simulink model "LQG_test"  (R2015a)
settings: Solver=ode5  StartTime=0.0  StopTime=14  FixedStep=1e-4  RelTol=1e-3
values from neighbouring files (symbols this model uses):
  Ak = [-64 -2560.5889522 8 186.2855092 1 -591.3291744 0 -1454.0827616 8 -3098.4577974 -142 -18500.7928836 ... (16 elements, 4x4)]    [controller.mat]    (also in main_matlab_step1.m = A-B*K-L*C)
  Ap = A(1:nn,1:nn)    [main_matlab_step1.m]    (also in plant.mat = [0 -330.46 0 -812.61 1 -12.15 0 -29.87 0 -2.44 0 -30.1 ... ()
  Bk = [64  -8; 2054  -280; -8  142; -1432  10169]    [controller.mat]    (also in main_matlab_step1.m = L)
  Bp = B    [main_matlab_step1.m]    (also in plant.mat = [0 2.71762 0 6.68268])
  Ck = [-64.81 -213.12 -1242.27 -85.82]    [controller.mat]    (also in main_matlab_step1.m = -K)
  Cp = C    [main_matlab_step1.m]    (also in plant.mat = [1  0  0  0; 0  0  1  0])
  Dk = [0 0]    [controller.mat]    (also in main_matlab_step1.m = zeros(1,2))
  Hp = H    [main_matlab_step1.m]    (also in plant.mat = [0 0 0 15.61])
libraries: simulink x1
settings Model: Creator=p4wp4w  LastModifiedBy=p4wp4w

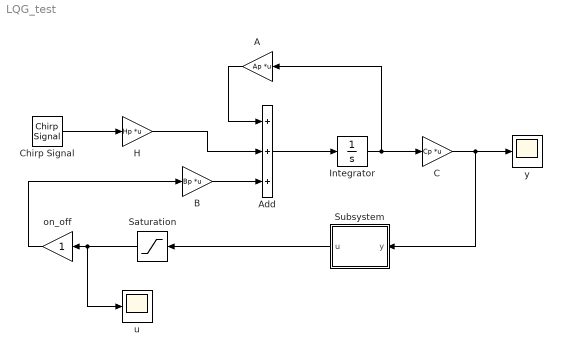
== system LQG_test ==
  A : Gain  Gain=Ap  Multiplication=Matrix(K*u)
  Add : Sum  Inputs=+++
  B : Gain  Gain=Bp  Multiplication=Matrix(K*u)
  C : Gain  Gain=Cp  Multiplication=Matrix(K*u)
  Chirp Signal : simulink/Sources/Chirp Signal  f1=0.1  T=14  f2=140
  H : Gain  Gain=Hp  Multiplication=Matrix(K*u)
  Integrator : Integrator
  Saturation : Saturate  UpperLimit=1.5  LowerLimit=-1.5
  Subsystem : Subsystem
  on_off : Gain
  u : Scope
      settings: YMin=-0.03  YMax=0.03
  y : Scope
      settings: YMin=-0.03  YMax=0.03
  wires:
  Add/1 -> Integrator/1
  A/1 -> Add/1
  B/1 -> Add/3
  Integrator/1 -> C/1, A/1
  H/1 -> Add/2
  Chirp Signal/1 -> H/1
  on_off/1 -> B/1
  Saturation/1 -> u/1, on_off/1
  C/1 -> Subsystem/1(y), y/1
  Subsystem/1("u ") -> Saturation/1

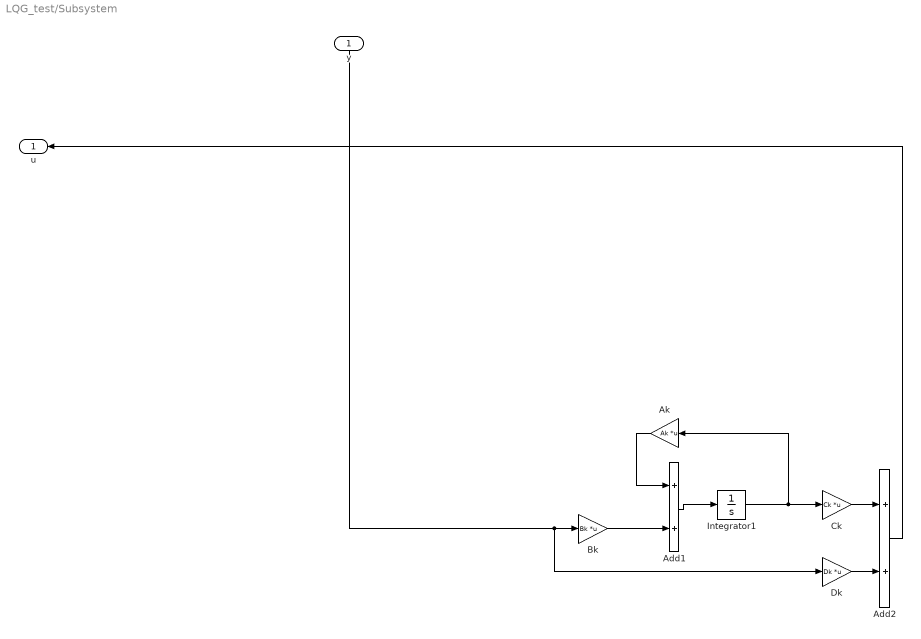
== system LQG_test/Subsystem ==
  y : Inport
  Add1 : Sum
  Add2 : Sum
  Ak : Gain  Gain=Ak  Multiplication=Matrix(K*u)
  Bk : Gain  Gain=Bk  Multiplication=Matrix(K*u)
  Ck : Gain  Gain=Ck  Multiplication=Matrix(K*u)
  Dk : Gain  Gain=Dk  Multiplication=Matrix(K*u)
  Integrator1 : Integrator
  "u " : Outport
  wires:
  y/1 -> Bk/1, Dk/1
  Add2/1 -> "u "/1
  Bk/1 -> Add1/2
  Ak/1 -> Add1/1
  Add1/1 -> Integrator1/1
  Dk/1 -> Add2/2
  Integrator1/1 -> Ck/1, Ak/1
  Ck/1 -> Add2/1
